simulink model "LoFT_Example3"  (R2024b)
settings: Solver=ode4  StartTime=0.0  StopTime=300  FixedStep=simu.dt  RelTol=1e-3
undefined symbols (not defined in the file): body, circtime, Communication, D1, Delta, irkb, line, LoFT, p0, Pn, s, simu, trip_time, Turbwind, waves, wind
libraries: simulink x350, spsThreePhaseVIMeasurementLib x41, spsThreePhasePISectionLineLib x34, spsThreePhaseParallelRLCLoadLib x21, spsThreePhaseTransformerTwoWindingsLib x14, spsLoadFlowBusLib x10, spsThreePhaseDynamicLoadLib x9, spsSynchronousMachinepuStandardLib x7, spsExcitationSystemLib x7, spsSteamTurbineandGovernorLib x7, spsGenericPowerSystemStabilizerLib x7, spsMultiBandPowerSystemStabilizerLib x7
(part 1 of 49)
settings Model: SimulationMode=accelerator  Creator=85164  LastModifiedBy=85164
settings DataIOCC: ReturnWorkspaceOutputs=off
settings OptimizationCC: ReuseModelBlockBuffer=off
settings RTWCC: GPUComputeCapability=3.5

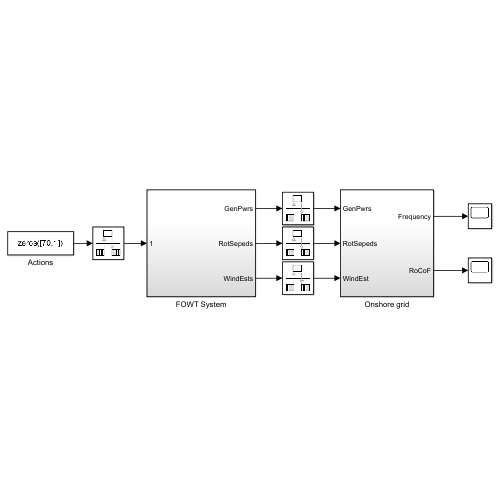
[thumbnail: Simulink's stored preview of the top-level diagram]
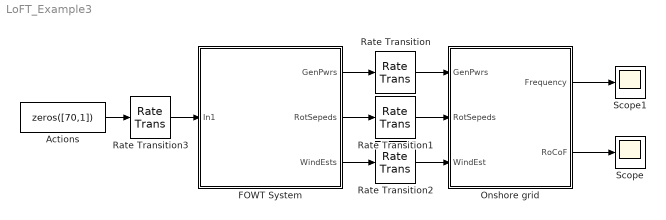
== system LoFT_Example3 ==
  Actions : Constant  Value=zeros([70,1])
  FOWT System : Subsystem
  Onshore grid : Subsystem
  Rate Transition : RateTransition  OutPortSampleTime=simu.grid_dt
  Rate Transition1 : RateTransition  OutPortSampleTime=simu.grid_dt
  Rate Transition2 : RateTransition  OutPortSampleTime=simu.grid_dt
  Rate Transition3 : RateTransition  OutPortSampleTime=simu.turbine_dt
  Scope : Scope
  Scope1 : Scope
  wires:
  FOWT System/1(GenPwrs) -> Rate Transition/1
  FOWT System/2(RotSepeds) -> Rate Transition1/1
  FOWT System/3(WindEsts) -> Rate Transition2/1
  Actions/1 -> Rate Transition3/1
  Onshore grid/1(Frequency) -> Scope1/1
  Onshore grid/2(RoCoF) -> Scope/1
  Rate Transition/1 -> Onshore grid/1(GenPwrs)
  Rate Transition1/1 -> Onshore grid/2(RotSepeds)
  Rate Transition2/1 -> Onshore grid/3(WindEst)
  Rate Transition3/1 -> FOWT System/1(In1)

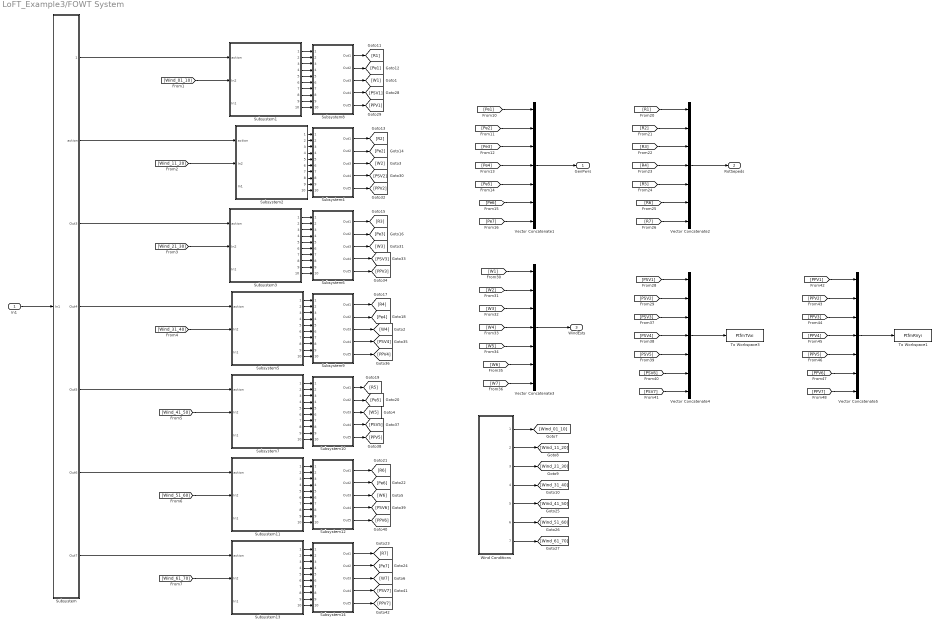
== system LoFT_Example3/FOWT System ==
  In1 : Inport
  Subsystem : Subsystem
  Subsystem1 : Subsystem
  Subsystem10 : Subsystem
  Subsystem11 : Subsystem
  Subsystem12 : Subsystem
  Subsystem13 : Subsystem
  Subsystem14 : Subsystem
  Subsystem2 : Subsystem
  Subsystem3 : Subsystem
  Subsystem4 : Subsystem
  Subsystem5 : Subsystem
  Subsystem6 : Subsystem
  Subsystem7 : Subsystem
  Subsystem8 : Subsystem
  Subsystem9 : Subsystem
  To Workspace1 : ToWorkspace  VariableName=PtfmRVyi  SampleTime=-1
      settings: Save2DSignal=2-D array (concatenate along first dimension)
  To Workspace3 : ToWorkspace  VariableName=PtfmTVxi  SampleTime=-1
      settings: Save2DSignal=2-D array (concatenate along first dimension)
  Vector Concatenate{1..5} (5 alike) : Concatenate  NumInputs=7
  Wind Conditions : Subsystem
  GenPwrs : Outport
  RotSepeds : Outport  Port=2
  WindEsts : Outport  Port=3
  wires:
  [Pe4] -> Vector Concatenate1/4
  [Pe1] -> Vector Concatenate1/1
  [Pe5] -> Vector Concatenate1/5
  [Pe3] -> Vector Concatenate1/3
  [Pe7] -> Vector Concatenate1/7
  [Pe2] -> Vector Concatenate1/2
  [Pe6] -> Vector Concatenate1/6
  [R2] -> Vector Concatenate2/2
  [R3] -> Vector Concatenate2/3
  [R4] -> Vector Concatenate2/4
  [R7] -> Vector Concatenate2/7
  [R5] -> Vector Concatenate2/5
  [R6] -> Vector Concatenate2/6
  [R1] -> Vector Concatenate2/1
  Vector Concatenate1/1 -> GenPwrs/1
  Vector Concatenate2/1 -> RotSepeds/1
  Subsystem/1(1) -> Subsystem1/1(action)
  Vector Concatenate3/1 -> WindEsts/1
  [W5] -> Vector Concatenate3/5
  [W3] -> Vector Concatenate3/3
  [W2] -> Vector Concatenate3/2
  [W1] -> Vector Concatenate3/1
  [W6] -> Vector Concatenate3/6
  [W7] -> Vector Concatenate3/7
  [W4] -> Vector Concatenate3/4
  Wind Conditions/1(1) -> [Wind_01_10]
  Wind Conditions/2(2) -> [Wind_11_20]
  Wind Conditions/3(3) -> [Wind_21_30]
  Wind Conditions/4(4) -> [Wind_31_40]
  Wind Conditions/5(5) -> [Wind_41_50]
  Wind Conditions/6(6) -> [Wind_51_60]
  Wind Conditions/7(7) -> [Wind_61_70]
  [Wind_01_10] -> Subsystem1/2(In2)
  [Wind_11_20] -> Subsystem2/2(In2)
  Subsystem/2(action) -> Subsystem2/1(action)
  [Wind_21_30] -> Subsystem3/2(In2)
  Subsystem/3(Out3) -> Subsystem3/1(action)
  Subsystem/4(Out4) -> Subsystem5/1(action)
  [Wind_31_40] -> Subsystem5/2(In2)
  Subsystem/5(Out5) -> Subsystem7/1(action)
  [Wind_41_50] -> Subsystem7/2(In2)
  Subsystem/6(Out6) -> Subsystem11/1(action)
  [Wind_51_60] -> Subsystem11/2(In2)
  [Wind_61_70] -> Subsystem13/2(In2)
  Subsystem/7(Out7) -> Subsystem13/1(action)
  In1/1 -> Subsystem/1(In1)
  Subsystem4/4(Out4) -> [PSV2]
  Subsystem13/4(4) -> Subsystem14/4(4)
  Subsystem8/3(Out3) -> [W1]
  Subsystem1/10(10) -> Subsystem8/10(10)
  Subsystem12/2(Out2) -> [Pe6]
  Subsystem1/7(7) -> Subsystem8/7(7)
  Subsystem10/2(Out2) -> [Pe5]
  Subsystem12/5(Out5) -> [PPV6]
  Subsystem14/4(Out4) -> [PSV7]
  Subsystem14/2(Out2) -> [Pe7]
  Subsystem4/2(Out2) -> [Pe2]
  Subsystem10/4(Out4) -> [PSV5]
  Subsystem9/2(Out2) -> [Pe4]
  Subsystem11/9(9) -> Subsystem12/9(9)
  Subsystem2/2(2) -> Subsystem4/2(2)
  Subsystem9/4(Out4) -> [PSV4]
  Subsystem13/6(6) -> Subsystem14/6(6)
  Subsystem12/4(Out4) -> [PSV6]
  Subsystem3/8(8) -> Subsystem6/8(8)
  Subsystem7/8(8) -> Subsystem10/8(8)
  Subsystem5/10(10) -> Subsystem9/10(10)
  Subsystem5/7(7) -> Subsystem9/7(7)
  Subsystem4/5(Out5) -> [PPV2]
  Subsystem8/5(Out5) -> [PPV1]
  Subsystem11/4(4) -> Subsystem12/4(4)
  Subsystem9/1(Out1) -> [R4]
  Subsystem4/1(Out1) -> [R2]
  Subsystem6/2(Out2) -> [Pe3]
  Subsystem12/1(Out1) -> [R6]
  Subsystem10/1(Out1) -> [R5]
  Subsystem8/4(Out4) -> [PSV1]
  Subsystem9/3(Out3) -> [W4]
  Subsystem11/6(6) -> Subsystem12/6(6)
  Subsystem14/1(Out1) -> [R7]
  Subsystem5/3(3) -> Subsystem9/3(3)
  Subsystem13/5(5) -> Subsystem14/5(5)
  Subsystem13/9(9) -> Subsystem14/9(9)
  Subsystem6/1(Out1) -> [R3]
  Subsystem11/2(2) -> Subsystem12/2(2)
  Subsystem7/4(4) -> Subsystem10/4(4)
  Subsystem3/4(4) -> Subsystem6/4(4)
  Subsystem11/7(7) -> Subsystem12/7(7)
  Subsystem13/10(10) -> Subsystem14/10(10)
  Subsystem7/2(2) -> Subsystem10/2(2)
  Subsystem2/3(3) -> Subsystem4/3(3)
  Subsystem7/1(1) -> Subsystem10/1(1)
  Subsystem11/10(10) -> Subsystem12/10(10)
  Subsystem7/9(9) -> Subsystem10/9(9)
  Subsystem1/2(2) -> Subsystem8/2(2)
  Subsystem7/3(3) -> Subsystem10/3(3)
  Subsystem5/5(5) -> Subsystem9/5(5)
  Subsystem11/8(8) -> Subsystem12/8(8)
  Subsystem5/8(8) -> Subsystem9/8(8)
  Subsystem3/3(3) -> Subsystem6/3(3)
  Subsystem11/1(1) -> Subsystem12/1(1)
  Subsystem3/5(5) -> Subsystem6/5(5)
  Subsystem5/6(6) -> Subsystem9/6(6)
  Subsystem3/7(7) -> Subsystem6/7(7)
  Subsystem7/7(7) -> Subsystem10/7(7)
  Subsystem8/2(Out2) -> [Pe1]
  Subsystem11/5(5) -> Subsystem12/5(5)
  Subsystem5/4(4) -> Subsystem9/4(4)
  Subsystem6/4(Out4) -> [PSV3]
  Subsystem2/10(10) -> Subsystem4/10(10)
  Subsystem1/8(8) -> Subsystem8/8(8)
  Subsystem5/9(9) -> Subsystem9/9(9)
  Subsystem13/3(3) -> Subsystem14/3(3)
  Subsystem13/2(2) -> Subsystem14/2(2)
  Subsystem10/5(Out5) -> [PPV5]
  Subsystem13/7(7) -> Subsystem14/7(7)
  Subsystem12/3(Out3) -> [W6]
  Subsystem10/3(Out3) -> [W5]
  Subsystem13/8(8) -> Subsystem14/8(8)
  Subsystem3/9(9) -> Subsystem6/9(9)
  Subsystem3/1(1) -> Subsystem6/1(1)
  Subsystem1/6(6) -> Subsystem8/6(6)
  Subsystem2/8(8) -> Subsystem4/8(8)
  Subsystem1/9(9) -> Subsystem8/9(9)
  Subsystem2/4(4) -> Subsystem4/4(4)
  Subsystem2/9(9) -> Subsystem4/9(9)
  Subsystem6/5(Out5) -> [PPV3]
  Subsystem13/1(1) -> Subsystem14/1(1)
  Subsystem3/2(2) -> Subsystem6/2(2)
  Subsystem14/5(Out5) -> [PPV7]
  Subsystem2/1(1) -> Subsystem4/1(1)
  Subsystem14/3(Out3) -> [W7]
  Subsystem11/3(3) -> Subsystem12/3(3)
  Subsystem1/4(4) -> Subsystem8/4(4)
  Subsystem4/3(Out3) -> [W2]
  Subsystem5/2(2) -> Subsystem9/2(2)
  Subsystem2/7(7) -> Subsystem4/7(7)
  Subsystem2/6(6) -> Subsystem4/6(6)
  Subsystem3/6(6) -> Subsystem6/6(6)
  Subsystem5/1(1) -> Subsystem9/1(1)
  Subsystem1/5(5) -> Subsystem8/5(5)
  Subsystem7/10(10) -> Subsystem10/10(10)
  Subsystem8/1(Out1) -> [R1]
  Subsystem9/5(Out5) -> [PPV4]
  Subsystem2/5(5) -> Subsystem4/5(5)
  Subsystem6/3(Out3) -> [W3]
  Subsystem3/10(10) -> Subsystem6/10(10)
  Subsystem1/3(3) -> Subsystem8/3(3)
  Subsystem1/1(1) -> Subsystem8/1(1)
  Subsystem7/6(6) -> Subsystem10/6(6)
  Subsystem7/5(5) -> Subsystem10/5(5)
  [PSV5] -> Vector Concatenate4/5
  [PSV7] -> Vector Concatenate4/7
  Vector Concatenate4/1 -> To Workspace3/1
  [PPV7] -> Vector Concatenate5/7
  [PPV4] -> Vector Concatenate5/4
  [PPV6] -> Vector Concatenate5/6
  [PSV2] -> Vector Concatenate4/2
  [PSV6] -> Vector Concatenate4/6
  [PSV3] -> Vector Concatenate4/3
  [PPV2] -> Vector Concatenate5/2
  [PSV4] -> Vector Concatenate4/4
  [PPV5] -> Vector Concatenate5/5
  [PPV3] -> Vector Concatenate5/3
  [PPV1] -> Vector Concatenate5/1
  Vector Concatenate5/1 -> To Workspace1/1
  [PSV1] -> Vector Concatenate4/1

== system LoFT_Example3/Onshore grid ==
  GenPwrs : Inport
  RotSepeds : Inport  Port=2
  WindEst : Inport  Port=3
  Monitor : Subsystem
  Onshore Grid : Subsystem
  Frequency : Outport
  RoCoF : Outport  Port=2
  wires:
  RotSepeds/1 -> Monitor/2(RotSepeds)
  WindEst/1 -> Monitor/3(3)
  Onshore Grid/1(Frequency) -> Frequency/1
  Onshore Grid/2(RoCoF) -> RoCoF/1
  GenPwrs/1 -> Onshore Grid/1(1), Monitor/1(GenPwrs)

== system LoFT_Example3/FOWT System/Subsystem ==
  In1 : Inport
  Demux : Demux  Outputs=70
  Mux{,1..6} (7 alike) : Mux  Inputs=10
  1 : Outport
  action : Outport  Port=2
  Out3 : Outport  Port=3
  Out4 : Outport  Port=4
  Out5 : Outport  Port=5
  Out6 : Outport  Port=6
  Out7 : Outport  Port=7
  wires:
  Demux/25 -> Mux2/5
  Demux/42 -> Mux4/2
  Demux/37 -> Mux3/7
  Demux/6 -> Mux/6
  Demux/56 -> Mux5/6
  Demux/9 -> Mux/9
  Demux/36 -> Mux3/6
  Demux/52 -> Mux5/2
  Demux/67 -> Mux6/7
  Demux/13 -> Mux1/3
  Demux/61 -> Mux6/1
  Demux/55 -> Mux5/5
  Demux/47 -> Mux4/7
  Demux/8 -> Mux/8
  Demux/29 -> Mux2/9
  Demux/7 -> Mux/7
  Demux/68 -> Mux6/8
  Demux/59 -> Mux5/9
  Demux/60 -> Mux5/10
  Demux/39 -> Mux3/9
  Demux/58 -> Mux5/8
  Demux/62 -> Mux6/2
  Demux/53 -> Mux5/3
  Demux/20 -> Mux1/10
  Demux/54 -> Mux5/4
  Demux/23 -> Mux2/3
  Demux/51 -> Mux5/1
  Mux3/1 -> Out4/1
  Demux/38 -> Mux3/8
  Demux/57 -> Mux5/7
  Demux/63 -> Mux6/3
  Demux/27 -> Mux2/7
  Demux/15 -> Mux1/5
  Demux/19 -> Mux1/9
  Demux/49 -> Mux4/9
  Demux/28 -> Mux2/8
  Demux/32 -> Mux3/2
  Demux/65 -> Mux6/5
  Demux/43 -> Mux4/3
  Demux/45 -> Mux4/5
  Demux/41 -> Mux4/1
  Demux/11 -> Mux1/1
  Demux/30 -> Mux2/10
  Demux/46 -> Mux4/6
  Mux/1 -> 1/1
  Demux/5 -> Mux/5
  Demux/40 -> Mux3/10
  Demux/2 -> Mux/2
  Demux/44 -> Mux4/4
  Demux/3 -> Mux/3
  Demux/48 -> Mux4/8
  Demux/50 -> Mux4/10
  Demux/24 -> Mux2/4
  Demux/21 -> Mux2/1
  Demux/22 -> Mux2/2
  Demux/26 -> Mux2/6
  Mux6/1 -> Out7/1
  Demux/12 -> Mux1/2
  Demux/35 -> Mux3/5
  Demux/31 -> Mux3/1
  Demux/4 -> Mux/4
  Demux/33 -> Mux3/3
  Demux/34 -> Mux3/4
  Demux/10 -> Mux/10
  Demux/64 -> Mux6/4
  Demux/66 -> Mux6/6
  Demux/70 -> Mux6/10
  Demux/69 -> Mux6/9
  Demux/14 -> Mux1/4
  Demux/16 -> Mux1/6
  Demux/17 -> Mux1/7
  Demux/18 -> Mux1/8
  Demux/1 -> Mux/1
  Mux1/1 -> action/1
  Mux2/1 -> Out3/1
  Mux5/1 -> Out6/1
  Mux4/1 -> Out5/1
  In1/1 -> Demux/1

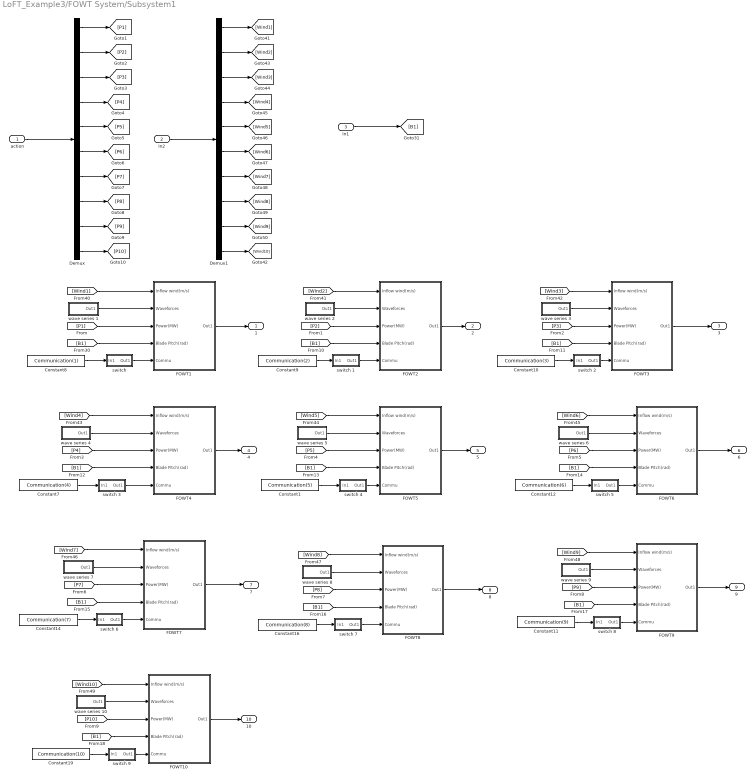
== system LoFT_Example3/FOWT System/Subsystem1 ==
  action : Inport
  In2 : Inport  Port=2
  In1 : Inport  Port=3
  Constant1 : Constant  Value=Communication(5)
  Constant10 : Constant  Value=Communication(3)
  Constant11 : Constant  Value=Communication(9)
  Constant12 : Constant  Value=Communication(6)
  Constant14 : Constant  Value=Communication(7)
  Constant16 : Constant  Value=Communication(8)
  Constant19 : Constant  Value=Communication(10)
  Constant7 : Constant  Value=Communication(4)
  Constant8 : Constant  Value=Communication(1)
  Constant9 : Constant  Value=Communication(2)
  Demux : Demux  Outputs=10
  Demux1 : Demux  Outputs=10
  FOWT1 : Subsystem  mask{Aero=LoFT.Aero, Hydro=LoFT.Hydro, Mooring=LoFT.Mooring, Property=LoFT.Property, Controller=LoFT.Controller, Initposition=[15,  0,  3*pi/180], Initstate=[6.8*pi/30, 9]}
      mask prompts: Aero "Aerodynamics"; Hydro "Hydrodynamics"; Mooring "Mooring lookup table"; Property "Hull mass, inertia and volume"; Controller "Local controller"; Initposition "Initial Hull position"; Initstate "Initial RotSpeed and WindEst"
      mask DialogControl DescGroupVar Prompt: LoFT
      mask DialogControl FOWT Prompt: Low-order modelling of floating offshore wind turbine for training
      mask DialogControl Manuscript Prompt: Citation
      mask DialogControl scriptname Prompt: Primary Frequency Response of Floating Offshore Wind Turbines via Deep Reinforcement Learning and Domain Randomization
      mask DialogControl ParameterGroupVar Prompt: 参数
  FOWT10 : Subsystem  mask{Aero=LoFT.Aero, Hydro=LoFT.Hydro, Mooring=LoFT.Mooring, Property=LoFT.Property, Controller=LoFT.Controller, Initposition=[5,  0,  3*pi/180], Initstate=[6.8*pi/30, 9]}
      mask prompts: Aero "Aerodynamics"; Hydro "Hydrodynamics"; Mooring "Mooring lookup table"; Property "Hull mass, inertia and volume"; Controller "Local controller"; Initposition "Initial Hull position"; Initstate "Initial RotSpeed and WindEst"
      mask DialogControl DescGroupVar Prompt: LoFT
      mask DialogControl FOWT Prompt: Low-order modelling of floating offshore wind turbine for training
      mask DialogControl Manuscript Prompt: Citation
      mask DialogControl scriptname Prompt: Primary Frequency Response of Floating Offshore Wind Turbines via Deep Reinforcement Learning and Domain Randomization
      mask DialogControl ParameterGroupVar Prompt: 参数
  FOWT2 : Subsystem  mask{Aero=LoFT.Aero, Hydro=LoFT.Hydro, Mooring=LoFT.Mooring, Property=LoFT.Property, Controller=LoFT.Controller, Initposition=[40,  0,  3*pi/180], Initstate=[6.8*pi/30, 9]}
      mask prompts: Aero "Aerodynamics"; Hydro "Hydrodynamics"; Mooring "Mooring lookup table"; Property "Hull mass, inertia and volume"; Controller "Local controller"; Initposition "Initial Hull position"; Initstate "Initial RotSpeed and WindEst"
      mask DialogControl DescGroupVar Prompt: LoFT
      mask DialogControl FOWT Prompt: Low-order modelling of floating offshore wind turbine for training
      mask DialogControl Manuscript Prompt: Citation
      mask DialogControl scriptname Prompt: Primary Frequency Response of Floating Offshore Wind Turbines via Deep Reinforcement Learning and Domain Randomization
      mask DialogControl ParameterGroupVar Prompt: 参数
  FOWT3 : Subsystem  mask{Aero=LoFT.Aero, Hydro=LoFT.Hydro, Mooring=LoFT.Mooring, Property=LoFT.Property, Controller=LoFT.Controller, Initposition=[25,  0,  3*pi/180], Initstate=[6.8*pi/30, 9]}
      mask prompts: Aero "Aerodynamics"; Hydro "Hydrodynamics"; Mooring "Mooring lookup table"; Property "Hull mass, inertia and volume"; Controller "Local controller"; Initposition "Initial Hull position"; Initstate "Initial RotSpeed and WindEst"
      mask DialogControl DescGroupVar Prompt: LoFT
      mask DialogControl FOWT Prompt: Low-order modelling of floating offshore wind turbine for training
      mask DialogControl Manuscript Prompt: Citation
      mask DialogControl scriptname Prompt: Primary Frequency Response of Floating Offshore Wind Turbines via Deep Reinforcement Learning and Domain Randomization
      mask DialogControl ParameterGroupVar Prompt: 参数
  FOWT4 : Subsystem  mask{Aero=LoFT.Aero, Hydro=LoFT.Hydro, Mooring=LoFT.Mooring, Property=LoFT.Property, Controller=LoFT.Controller, Initposition=[15,  0,  3*pi/180], Initstate=[6.8*pi/30, 9]}
      mask prompts: Aero "Aerodynamics"; Hydro "Hydrodynamics"; Mooring "Mooring lookup table"; Property "Hull mass, inertia and volume"; Controller "Local controller"; Initposition "Initial Hull position"; Initstate "Initial RotSpeed and WindEst"
      mask DialogControl DescGroupVar Prompt: LoFT
      mask DialogControl FOWT Prompt: Low-order modelling of floating offshore wind turbine for training
      mask DialogControl Manuscript Prompt: Citation
      mask DialogControl scriptname Prompt: Primary Frequency Response of Floating Offshore Wind Turbines via Deep Reinforcement Learning and Domain Randomization
      mask DialogControl ParameterGroupVar Prompt: 参数
  FOWT5 : Subsystem  mask{Aero=LoFT.Aero, Hydro=LoFT.Hydro, Mooring=LoFT.Mooring, Property=LoFT.Property, Controller=LoFT.Controller, Initposition=[40,  0,  3*pi/180], Initstate=[6.8*pi/30, 9]}
      mask prompts: Aero "Aerodynamics"; Hydro "Hydrodynamics"; Mooring "Mooring lookup table"; Property "Hull mass, inertia and volume"; Controller "Local controller"; Initposition "Initial Hull position"; Initstate "Initial RotSpeed and WindEst"
      mask DialogControl DescGroupVar Prompt: LoFT
      mask DialogControl FOWT Prompt: Low-order modelling of floating offshore wind turbine for training
      mask DialogControl Manuscript Prompt: Citation
      mask DialogControl scriptname Prompt: Primary Frequency Response of Floating Offshore Wind Turbines via Deep Reinforcement Learning and Domain Randomization
      mask DialogControl ParameterGroupVar Prompt: 参数
  FOWT6 : Subsystem  mask{Aero=LoFT.Aero, Hydro=LoFT.Hydro, Mooring=LoFT.Mooring, Property=LoFT.Property, Controller=LoFT.Controller, Initposition=[25,  0,  3*pi/180], Initstate=[6.8*pi/30, 9]}
      mask prompts: Aero "Aerodynamics"; Hydro "Hydrodynamics"; Mooring "Mooring lookup table"; Property "Hull mass, inertia and volume"; Controller "Local controller"; Initposition "Initial Hull position"; Initstate "Initial RotSpeed and WindEst"
      mask DialogControl DescGroupVar Prompt: LoFT
      mask DialogControl FOWT Prompt: Low-order modelling of floating offshore wind turbine for training
      mask DialogControl Manuscript Prompt: Citation
      mask DialogControl scriptname Prompt: Primary Frequency Response of Floating Offshore Wind Turbines via Deep Reinforcement Learning and Domain Randomization
      mask DialogControl ParameterGroupVar Prompt: 参数
  FOWT7 : Subsystem  mask{Aero=LoFT.Aero, Hydro=LoFT.Hydro, Mooring=LoFT.Mooring, Property=LoFT.Property, Controller=LoFT.Controller, Initposition=[15,  0,  3*pi/180], Initstate=[6.8*pi/30, 9]}
      mask prompts: Aero "Aerodynamics"; Hydro "Hydrodynamics"; Mooring "Mooring lookup table"; Property "Hull mass, inertia and volume"; Controller "Local controller"; Initposition "Initial Hull position"; Initstate "Initial RotSpeed and WindEst"
      mask DialogControl DescGroupVar Prompt: LoFT
      mask DialogControl FOWT Prompt: Low-order modelling of floating offshore wind turbine for training
      mask DialogControl Manuscript Prompt: Citation
      mask DialogControl scriptname Prompt: Primary Frequency Response of Floating Offshore Wind Turbines via Deep Reinforcement Learning and Domain Randomization
      mask DialogControl ParameterGroupVar Prompt: 参数
  FOWT8 : Subsystem  mask{Aero=LoFT.Aero, Hydro=LoFT.Hydro, Mooring=LoFT.Mooring, Property=LoFT.Property, Controller=LoFT.Controller, Initposition=[40,  0,  3*pi/180], Initstate=[6.8*pi/30, 9]}
      mask prompts: Aero "Aerodynamics"; Hydro "Hydrodynamics"; Mooring "Mooring lookup table"; Property "Hull mass, inertia and volume"; Controller "Local controller"; Initposition "Initial Hull position"; Initstate "Initial RotSpeed and WindEst"
      mask DialogControl DescGroupVar Prompt: LoFT
      mask DialogControl FOWT Prompt: Low-order modelling of floating offshore wind turbine for training
      mask DialogControl Manuscript Prompt: Citation
      mask DialogControl scriptname Prompt: Primary Frequency Response of Floating Offshore Wind Turbines via Deep Reinforcement Learning and Domain Randomization
      mask DialogControl ParameterGroupVar Prompt: 参数
  FOWT9 : Subsystem  mask{Aero=LoFT.Aero, Hydro=LoFT.Hydro, Mooring=LoFT.Mooring, Property=LoFT.Property, Controller=LoFT.Controller, Initposition=[25,  0,  3*pi/180], Initstate=[6.8*pi/30, 9]}
      mask prompts: Aero "Aerodynamics"; Hydro "Hydrodynamics"; Mooring "Mooring lookup table"; Property "Hull mass, inertia and volume"; Controller "Local controller"; Initposition "Initial Hull position"; Initstate "Initial RotSpeed and WindEst"
      mask DialogControl DescGroupVar Prompt: LoFT
      mask DialogControl FOWT Prompt: Low-order modelling of floating offshore wind turbine for training
      mask DialogControl Manuscript Prompt: Citation
      mask DialogControl scriptname Prompt: Primary Frequency Response of Floating Offshore Wind Turbines via Deep Reinforcement Learning and Domain Randomization
      mask DialogControl ParameterGroupVar Prompt: 参数
  "switch " : Subsystem
  switch 1 : Subsystem
  switch 2 : Subsystem
  switch 3 : Subsystem
  switch 4 : Subsystem
  switch 5 : Subsystem
  switch 6 : Subsystem
  switch 7 : Subsystem
  switch 8 : Subsystem
  switch 9 : Subsystem
  wave series 1 : Subsystem
  wave series 10 : Subsystem
  wave series 2 : Subsystem
  wave series 3 : Subsystem
  wave series 4 : Subsystem
  wave series 5 : Subsystem
  wave series 6 : Subsystem
  wave series 7 : Subsystem
  wave series 8 : Subsystem
  wave series 9 : Subsystem
  1 : Outport
  2 : Outport  Port=2
  3 : Outport  Port=3
  4 : Outport  Port=4
  5 : Outport  Port=5
  6 : Outport  Port=6
  7 : Outport  Port=7
  8 : Outport  Port=8
  9 : Outport  Port=9
  10 : Outport  Port=10
  wires:
  Demux/9 -> [P9]
  Demux/10 -> [P10]
  wave series 10/1(Out1) -> FOWT10/2(Waveforces)
  [B1] -> FOWT10/4(Blade Pitch(rad))
  Constant19/1 -> switch 9/1(In1)
  switch 9/1(Out1) -> FOWT10/5(Commu)
  [P10] -> FOWT10/3(Power(MW))
  [Wind10] -> FOWT10/1(Inflow wind(m/s))
  Constant11/1 -> switch 8/1(In1)
  [P9] -> FOWT9/3(Power(MW))
  [B1] -> FOWT9/4(Blade Pitch(rad))
  [Wind9] -> FOWT9/1(Inflow wind(m/s))
  switch 8/1(Out1) -> FOWT9/5(Commu)
  wave series 9/1(Out1) -> FOWT9/2(Waveforces)
  Demux/6 -> [P6]
  Demux/7 -> [P7]
  Demux/8 -> [P8]
  Demux/5 -> [P5]
  Demux/1 -> [P1]
  Demux/4 -> [P4]
  action/1 -> Demux/1
  Demux/3 -> [P3]
  Demux/2 -> [P2]
  [Wind2] -> FOWT2/1(Inflow wind(m/s))
  wave series 2/1(Out1) -> FOWT2/2(Waveforces)
  [Wind4] -> FOWT4/1(Inflow wind(m/s))
  wave series 8/1(Out1) -> FOWT8/2(Waveforces)
  [Wind3] -> FOWT3/1(Inflow wind(m/s))
  switch 4/1(Out1) -> FOWT5/5(Commu)
  switch 7/1(Out1) -> FOWT8/5(Commu)
  wave series 4/1(Out1) -> FOWT4/2(Waveforces)
  switch 6/1(Out1) -> FOWT7/5(Commu)
  Constant16/1 -> switch 7/1(In1)
  wave series 6/1(Out1) -> FOWT6/2(Waveforces)
  [Wind8] -> FOWT8/1(Inflow wind(m/s))
  wave series 1/1(Out1) -> FOWT1/2(Waveforces)
  [Wind5] -> FOWT5/1(Inflow wind(m/s))
  Constant8/1 -> "switch "/1(In1)
  "switch "/1(Out1) -> FOWT1/5(Commu)
  [P8] -> FOWT8/3(Power(MW))
  [B1] -> FOWT8/4(Blade Pitch(rad))
  wave series 5/1(Out1) -> FOWT5/2(Waveforces)
  Constant10/1 -> switch 2/1(In1)
  [P5] -> FOWT5/3(Power(MW))
  Constant14/1 -> switch 6/1(In1)
  [P6] -> FOWT6/3(Power(MW))
  Constant12/1 -> switch 5/1(In1)
  [P4] -> FOWT4/3(Power(MW))
  wave series 7/1(Out1) -> FOWT7/2(Waveforces)
  [Wind7] -> FOWT7/1(Inflow wind(m/s))
  [P1] -> FOWT1/3(Power(MW))
  [B1] -> FOWT7/4(Blade Pitch(rad))
  [P3] -> FOWT3/3(Power(MW))
  Constant1/1 -> switch 4/1(In1)
  switch 1/1(Out1) -> FOWT2/5(Commu)
  [Wind1] -> FOWT1/1(Inflow wind(m/s))
  [P2] -> FOWT2/3(Power(MW))
  [Wind6] -> FOWT6/1(Inflow wind(m/s))
  wave series 3/1(Out1) -> FOWT3/2(Waveforces)
  Constant7/1 -> switch 3/1(In1)
  Constant9/1 -> switch 1/1(In1)
  [P7] -> FOWT7/3(Power(MW))
  switch 5/1(Out1) -> FOWT6/5(Commu)
  switch 3/1(Out1) -> FOWT4/5(Commu)
  switch 2/1(Out1) -> FOWT3/5(Commu)
  Demux1/4 -> [Wind4]
  In2/1 -> Demux1/1
  Demux1/7 -> [Wind7]
  Demux1/8 -> [Wind8]
  Demux1/3 -> [Wind3]
  Demux1/2 -> [Wind2]
  Demux1/5 -> [Wind5]
  Demux1/9 -> [Wind9]
  Demux1/10 -> [Wind10]
  Demux1/1 -> [Wind1]
  Demux1/6 -> [Wind6]
  FOWT1/1(Out1) -> 1/1
  FOWT2/1(Out1) -> 2/1
  FOWT3/1(Out1) -> 3/1
  FOWT4/1(Out1) -> 4/1
  FOWT5/1(Out1) -> 5/1
  FOWT6/1(Out1) -> 6/1
  FOWT7/1(Out1) -> 7/1
  FOWT8/1(Out1) -> 8/1
  FOWT9/1(Out1) -> 9/1
  FOWT10/1(Out1) -> 10/1
  In1/1 -> [B1]
  [B1] -> FOWT1/4(Blade Pitch(rad))
  [B1] -> FOWT2/4(Blade Pitch(rad))
  [B1] -> FOWT3/4(Blade Pitch(rad))
  [B1] -> FOWT4/4(Blade Pitch(rad))
  [B1] -> FOWT5/4(Blade Pitch(rad))
  [B1] -> FOWT6/4(Blade Pitch(rad))

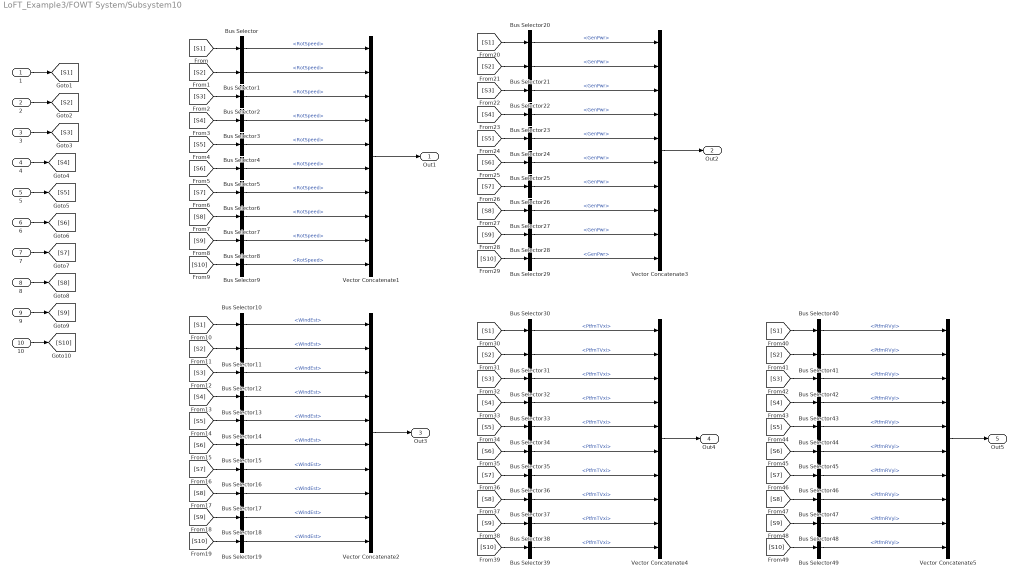
== system LoFT_Example3/FOWT System/Subsystem10 ==
  1 : Inport
  2 : Inport  Port=2
  3 : Inport  Port=3
  4 : Inport  Port=4
  5 : Inport  Port=5
  6 : Inport  Port=6
  7 : Inport  Port=7
  8 : Inport  Port=8
  9 : Inport  Port=9
  10 : Inport  Port=10
  Bus Selector{,1..9} (10 alike) : BusSelector  OutputSignals=RotSpeed
  Bus Selector{10..19} (10 alike) : BusSelector  OutputSignals=WindEst
  Bus Selector{20..29} (10 alike) : BusSelector  OutputSignals=GenPwr
  Bus Selector{30..39} (10 alike) : BusSelector  OutputSignals=PtfmTVxi
  Bus Selector{40..49} (10 alike) : BusSelector  OutputSignals=PtfmRVyi
  Vector Concatenate{1..5} (5 alike) : Concatenate  NumInputs=10
  Out1 : Outport
  Out2 : Outport  Port=2
  Out3 : Outport  Port=3
  Out4 : Outport  Port=4
  Out5 : Outport  Port=5
  wires:
  1/1 -> [S1]
  2/1 -> [S2]
  3/1 -> [S3]
  4/1 -> [S4]
  5/1 -> [S5]
  6/1 -> [S6]
  7/1 -> [S7]
  8/1 -> [S8]
  9/1 -> [S9]
  10/1 -> [S10]
  [S1] -> Bus Selector/1
  Vector Concatenate1/1 -> Out1/1
  Bus Selector/1 -> Vector Concatenate1/1  "<RotSpeed>"
  [S2] -> Bus Selector1/1
  Bus Selector1/1 -> Vector Concatenate1/2  "<RotSpeed>"
  Bus Selector2/1 -> Vector Concatenate1/3  "<RotSpeed>"
  [S3] -> Bus Selector2/1
  [S4] -> Bus Selector3/1
  Bus Selector3/1 -> Vector Concatenate1/4  "<RotSpeed>"
  [S5] -> Bus Selector4/1
  [S6] -> Bus Selector5/1
  [S7] -> Bus Selector6/1
  [S8] -> Bus Selector7/1
  [S9] -> Bus Selector8/1
  [S10] -> Bus Selector9/1
  Bus Selector4/1 -> Vector Concatenate1/5  "<RotSpeed>"
  Bus Selector5/1 -> Vector Concatenate1/6  "<RotSpeed>"
  Bus Selector6/1 -> Vector Concatenate1/7  "<RotSpeed>"
  Bus Selector7/1 -> Vector Concatenate1/8  "<RotSpeed>"
  Bus Selector8/1 -> Vector Concatenate1/9  "<RotSpeed>"
  Bus Selector9/1 -> Vector Concatenate1/10  "<RotSpeed>"
  Bus Selector19/1 -> Vector Concatenate2/10  "<WindEst>"
  Bus Selector18/1 -> Vector Concatenate2/9  "<WindEst>"
  Bus Selector17/1 -> Vector Concatenate2/8  "<WindEst>"
  Bus Selector16/1 -> Vector Concatenate2/7  "<WindEst>"
  Bus Selector15/1 -> Vector Concatenate2/6  "<WindEst>"
  Bus Selector14/1 -> Vector Concatenate2/5  "<WindEst>"
  [S10] -> Bus Selector19/1
  [S9] -> Bus Selector18/1
  [S7] -> Bus Selector16/1
  [S6] -> Bus Selector15/1
  [S5] -> Bus Selector14/1
  Bus Selector13/1 -> Vector Concatenate2/4  "<WindEst>"
  [S4] -> Bus Selector13/1
  [S3] -> Bus Selector12/1
  Bus Selector12/1 -> Vector Concatenate2/3  "<WindEst>"
  Bus Selector11/1 -> Vector Concatenate2/2  "<WindEst>"
  [S2] -> Bus Selector11/1
  Bus Selector10/1 -> Vector Concatenate2/1  "<WindEst>"
  [S1] -> Bus Selector10/1
  [S1] -> Bus Selector20/1
  Bus Selector20/1 -> Vector Concatenate3/1  "<GenPwr>"
  [S2] -> Bus Selector21/1
  Bus Selector21/1 -> Vector Concatenate3/2  "<GenPwr>"
  Bus Selector22/1 -> Vector Concatenate3/3  "<GenPwr>"
  [S3] -> Bus Selector22/1
  [S4] -> Bus Selector23/1
  Bus Selector23/1 -> Vector Concatenate3/4  "<GenPwr>"
  [S5] -> Bus Selector24/1
  [S6] -> Bus Selector25/1
  [S7] -> Bus Selector26/1
  [S8] -> Bus Selector27/1
  [S9] -> Bus Selector28/1
  [S10] -> Bus Selector29/1
  Bus Selector24/1 -> Vector Concatenate3/5  "<GenPwr>"
  Bus Selector25/1 -> Vector Concatenate3/6  "<GenPwr>"
  Bus Selector26/1 -> Vector Concatenate3/7  "<GenPwr>"
  Bus Selector27/1 -> Vector Concatenate3/8  "<GenPwr>"
  Bus Selector28/1 -> Vector Concatenate3/9  "<GenPwr>"
  Bus Selector29/1 -> Vector Concatenate3/10  "<GenPwr>"
  [S8] -> Bus Selector17/1
  Vector Concatenate3/1 -> Out2/1
  Vector Concatenate2/1 -> Out3/1
  [S1] -> Bus Selector30/1
  Bus Selector30/1 -> Vector Concatenate4/1  "<PtfmTVxi>"
  Vector Concatenate4/1 -> Out4/1
  [S5] -> Bus Selector44/1
  Bus Selector47/1 -> Vector Concatenate5/8  "<PtfmRVyi>"
  [S1] -> Bus Selector40/1
  Bus Selector40/1 -> Vector Concatenate5/1  "<PtfmRVyi>"
  [S2] -> Bus Selector41/1
  [S4] -> Bus Selector43/1
  [S3] -> Bus Selector42/1
  Bus Selector42/1 -> Vector Concatenate5/3  "<PtfmRVyi>"
  Bus Selector44/1 -> Vector Concatenate5/5  "<PtfmRVyi>"
  Bus Selector43/1 -> Vector Concatenate5/4  "<PtfmRVyi>"
  [S9] -> Bus Selector48/1
  Bus Selector45/1 -> Vector Concatenate5/6  "<PtfmRVyi>"
  Bus Selector48/1 -> Vector Concatenate5/9  "<PtfmRVyi>"
  [S6] -> Bus Selector45/1
  [S10] -> Bus Selector49/1
  Bus Selector49/1 -> Vector Concatenate5/10  "<PtfmRVyi>"
  Vector Concatenate5/1 -> Out5/1
  [S7] -> Bus Selector46/1
  Bus Selector46/1 -> Vector Concatenate5/7  "<PtfmRVyi>"
  Bus Selector41/1 -> Vector Concatenate5/2  "<PtfmRVyi>"
  [S8] -> Bus Selector47/1
  Bus Selector31/1 -> Vector Concatenate4/2  "<PtfmTVxi>"
  [S2] -> Bus Selector31/1
  Bus Selector32/1 -> Vector Concatenate4/3  "<PtfmTVxi>"
  [S3] -> Bus Selector32/1
  [S4] -> Bus Selector33/1
  Bus Selector33/1 -> Vector Concatenate4/4  "<PtfmTVxi>"
  [S5] -> Bus Selector34/1
  Bus Selector34/1 -> Vector Concatenate4/5  "<PtfmTVxi>"
  [S6] -> Bus Selector35/1
  Bus Selector35/1 -> Vector Concatenate4/6  "<PtfmTVxi>"
  [S7] -> Bus Selector36/1
  Bus Selector36/1 -> Vector Concatenate4/7  "<PtfmTVxi>"
  [S8] -> Bus Selector37/1
  Bus Selector37/1 -> Vector Concatenate4/8  "<PtfmTVxi>"
  [S9] -> Bus Selector38/1
  Bus Selector38/1 -> Vector Concatenate4/9  "<PtfmTVxi>"
  [S10] -> Bus Selector39/1
  Bus Selector39/1 -> Vector Concatenate4/10  "<PtfmTVxi>"

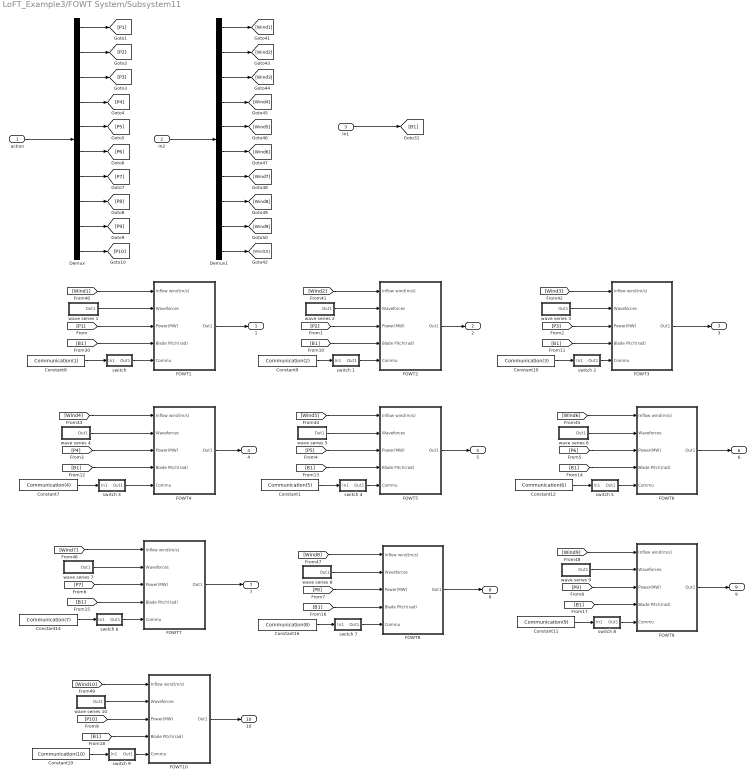
== system LoFT_Example3/FOWT System/Subsystem11 ==
  action : Inport
  In2 : Inport  Port=2
  In1 : Inport  Port=3
  Constant1 : Constant  Value=Communication(5)
  Constant10 : Constant  Value=Communication(3)
  Constant11 : Constant  Value=Communication(9)
  Constant12 : Constant  Value=Communication(6)
  Constant14 : Constant  Value=Communication(7)
  Constant16 : Constant  Value=Communication(8)
  Constant19 : Constant  Value=Communication(10)
  Constant7 : Constant  Value=Communication(4)
  Constant8 : Constant  Value=Communication(1)
  Constant9 : Constant  Value=Communication(2)
  Demux : Demux  Outputs=10
  Demux1 : Demux  Outputs=10
  FOWT1 : Subsystem  mask{Aero=LoFT.Aero, Hydro=LoFT.Hydro, Mooring=LoFT.Mooring, Property=LoFT.Property, Controller=LoFT.Controller, Initposition=[15,  0,  3*pi/180], Initstate=[6.8*pi/30, 9]}
      mask prompts: Aero "Aerodynamics"; Hydro "Hydrodynamics"; Mooring "Mooring lookup table"; Property "Hull mass, inertia and volume"; Controller "Local controller"; Initposition "Initial Hull position"; Initstate "Initial RotSpeed and WindEst"
      mask DialogControl DescGroupVar Prompt: LoFT
      mask DialogControl FOWT Prompt: Low-order modelling of floating offshore wind turbine for training
      mask DialogControl Manuscript Prompt: Citation
      mask DialogControl scriptname Prompt: Primary Frequency Response of Floating Offshore Wind Turbines via Deep Reinforcement Learning and Domain Randomization
      mask DialogControl ParameterGroupVar Prompt: 参数
  FOWT10 : Subsystem  mask{Aero=LoFT.Aero, Hydro=LoFT.Hydro, Mooring=LoFT.Mooring, Property=LoFT.Property, Controller=LoFT.Controller, Initposition=[5,  0,  3*pi/180], Initstate=[6.8*pi/30, 9]}
      mask prompts: Aero "Aerodynamics"; Hydro "Hydrodynamics"; Mooring "Mooring lookup table"; Property "Hull mass, inertia and volume"; Controller "Local controller"; Initposition "Initial Hull position"; Initstate "Initial RotSpeed and WindEst"
      mask DialogControl DescGroupVar Prompt: LoFT
      mask DialogControl FOWT Prompt: Low-order modelling of floating offshore wind turbine for training
      mask DialogControl Manuscript Prompt: Citation
      mask DialogControl scriptname Prompt: Primary Frequency Response of Floating Offshore Wind Turbines via Deep Reinforcement Learning and Domain Randomization
      mask DialogControl ParameterGroupVar Prompt: 参数
  FOWT2 : Subsystem  mask{Aero=LoFT.Aero, Hydro=LoFT.Hydro, Mooring=LoFT.Mooring, Property=LoFT.Property, Controller=LoFT.Controller, Initposition=[40,  0,  3*pi/180], Initstate=[6.8*pi/30, 9]}
      mask prompts: Aero "Aerodynamics"; Hydro "Hydrodynamics"; Mooring "Mooring lookup table"; Property "Hull mass, inertia and volume"; Controller "Local controller"; Initposition "Initial Hull position"; Initstate "Initial RotSpeed and WindEst"
      mask DialogControl DescGroupVar Prompt: LoFT
      mask DialogControl FOWT Prompt: Low-order modelling of floating offshore wind turbine for training
      mask DialogControl Manuscript Prompt: Citation
      mask DialogControl scriptname Prompt: Primary Frequency Response of Floating Offshore Wind Turbines via Deep Reinforcement Learning and Domain Randomization
      mask DialogControl ParameterGroupVar Prompt: 参数
  FOWT3 : Subsystem  mask{Aero=LoFT.Aero, Hydro=LoFT.Hydro, Mooring=LoFT.Mooring, Property=LoFT.Property, Controller=LoFT.Controller, Initposition=[25,  0,  3*pi/180], Initstate=[6.8*pi/30, 9]}
      mask prompts: Aero "Aerodynamics"; Hydro "Hydrodynamics"; Mooring "Mooring lookup table"; Property "Hull mass, inertia and volume"; Controller "Local controller"; Initposition "Initial Hull position"; Initstate "Initial RotSpeed and WindEst"
      mask DialogControl DescGroupVar Prompt: LoFT
      mask DialogControl FOWT Prompt: Low-order modelling of floating offshore wind turbine for training
      mask DialogControl Manuscript Prompt: Citation
      mask DialogControl scriptname Prompt: Primary Frequency Response of Floating Offshore Wind Turbines via Deep Reinforcement Learning and Domain Randomization
      mask DialogControl ParameterGroupVar Prompt: 参数
  FOWT4 : Subsystem  mask{Aero=LoFT.Aero, Hydro=LoFT.Hydro, Mooring=LoFT.Mooring, Property=LoFT.Property, Controller=LoFT.Controller, Initposition=[15,  0,  3*pi/180], Initstate=[6.8*pi/30, 9]}
      mask prompts: Aero "Aerodynamics"; Hydro "Hydrodynamics"; Mooring "Mooring lookup table"; Property "Hull mass, inertia and volume"; Controller "Local controller"; Initposition "Initial Hull position"; Initstate "Initial RotSpeed and WindEst"
      mask DialogControl DescGroupVar Prompt: LoFT
      mask DialogControl FOWT Prompt: Low-order modelling of floating offshore wind turbine for training
      mask DialogControl Manuscript Prompt: Citation
      mask DialogControl scriptname Prompt: Primary Frequency Response of Floating Offshore Wind Turbines via Deep Reinforcement Learning and Domain Randomization
      mask DialogControl ParameterGroupVar Prompt: 参数
  FOWT5 : Subsystem  mask{Aero=LoFT.Aero, Hydro=LoFT.Hydro, Mooring=LoFT.Mooring, Property=LoFT.Property, Controller=LoFT.Controller, Initposition=[40,  0,  3*pi/180], Initstate=[6.8*pi/30, 9]}
      mask prompts: Aero "Aerodynamics"; Hydro "Hydrodynamics"; Mooring "Mooring lookup table"; Property "Hull mass, inertia and volume"; Controller "Local controller"; Initposition "Initial Hull position"; Initstate "Initial RotSpeed and WindEst"
      mask DialogControl DescGroupVar Prompt: LoFT
      mask DialogControl FOWT Prompt: Low-order modelling of floating offshore wind turbine for training
      mask DialogControl Manuscript Prompt: Citation
      mask DialogControl scriptname Prompt: Primary Frequency Response of Floating Offshore Wind Turbines via Deep Reinforcement Learning and Domain Randomization
      mask DialogControl ParameterGroupVar Prompt: 参数
  FOWT6 : Subsystem  mask{Aero=LoFT.Aero, Hydro=LoFT.Hydro, Mooring=LoFT.Mooring, Property=LoFT.Property, Controller=LoFT.Controller, Initposition=[25,  0,  3*pi/180], Initstate=[6.8*pi/30, 9]}
      mask prompts: Aero "Aerodynamics"; Hydro "Hydrodynamics"; Mooring "Mooring lookup table"; Property "Hull mass, inertia and volume"; Controller "Local controller"; Initposition "Initial Hull position"; Initstate "Initial RotSpeed and WindEst"
      mask DialogControl DescGroupVar Prompt: LoFT
      mask DialogControl FOWT Prompt: Low-order modelling of floating offshore wind turbine for training
      mask DialogControl Manuscript Prompt: Citation
      mask DialogControl scriptname Prompt: Primary Frequency Response of Floating Offshore Wind Turbines via Deep Reinforcement Learning and Domain Randomization
      mask DialogControl ParameterGroupVar Prompt: 参数
  FOWT7 : Subsystem  mask{Aero=LoFT.Aero, Hydro=LoFT.Hydro, Mooring=LoFT.Mooring, Property=LoFT.Property, Controller=LoFT.Controller, Initposition=[15,  0,  3*pi/180], Initstate=[6.8*pi/30, 9]}
      mask prompts: Aero "Aerodynamics"; Hydro "Hydrodynamics"; Mooring "Mooring lookup table"; Property "Hull mass, inertia and volume"; Controller "Local controller"; Initposition "Initial Hull position"; Initstate "Initial RotSpeed and WindEst"
      mask DialogControl DescGroupVar Prompt: LoFT
      mask DialogControl FOWT Prompt: Low-order modelling of floating offshore wind turbine for training
      mask DialogControl Manuscript Prompt: Citation
      mask DialogControl scriptname Prompt: Primary Frequency Response of Floating Offshore Wind Turbines via Deep Reinforcement Learning and Domain Randomization
      mask DialogControl ParameterGroupVar Prompt: 参数
  FOWT8 : Subsystem  mask{Aero=LoFT.Aero, Hydro=LoFT.Hydro, Mooring=LoFT.Mooring, Property=LoFT.Property, Controller=LoFT.Controller, Initposition=[40,  0,  3*pi/180], Initstate=[6.8*pi/30, 9]}
      mask prompts: Aero "Aerodynamics"; Hydro "Hydrodynamics"; Mooring "Mooring lookup table"; Property "Hull mass, inertia and volume"; Controller "Local controller"; Initposition "Initial Hull position"; Initstate "Initial RotSpeed and WindEst"
      mask DialogControl DescGroupVar Prompt: LoFT
      mask DialogControl FOWT Prompt: Low-order modelling of floating offshore wind turbine for training
      mask DialogControl Manuscript Prompt: Citation
      mask DialogControl scriptname Prompt: Primary Frequency Response of Floating Offshore Wind Turbines via Deep Reinforcement Learning and Domain Randomization
      mask DialogControl ParameterGroupVar Prompt: 参数
  FOWT9 : Subsystem  mask{Aero=LoFT.Aero, Hydro=LoFT.Hydro, Mooring=LoFT.Mooring, Property=LoFT.Property, Controller=LoFT.Controller, Initposition=[25,  0,  3*pi/180], Initstate=[6.8*pi/30, 9]}
      mask prompts: Aero "Aerodynamics"; Hydro "Hydrodynamics"; Mooring "Mooring lookup table"; Property "Hull mass, inertia and volume"; Controller "Local controller"; Initposition "Initial Hull position"; Initstate "Initial RotSpeed and WindEst"
      mask DialogControl DescGroupVar Prompt: LoFT
      mask DialogControl FOWT Prompt: Low-order modelling of floating offshore wind turbine for training
      mask DialogControl Manuscript Prompt: Citation
      mask DialogControl scriptname Prompt: Primary Frequency Response of Floating Offshore Wind Turbines via Deep Reinforcement Learning and Domain Randomization
      mask DialogControl ParameterGroupVar Prompt: 参数
  "switch " : Subsystem
  switch 1 : Subsystem
  switch 2 : Subsystem
  switch 3 : Subsystem
  switch 4 : Subsystem
  switch 5 : Subsystem
  switch 6 : Subsystem
  switch 7 : Subsystem
  switch 8 : Subsystem
  switch 9 : Subsystem
  wave series 1 : Subsystem
  wave series 10 : Subsystem
  wave series 2 : Subsystem
  wave series 3 : Subsystem
  wave series 4 : Subsystem
  wave series 5 : Subsystem
  wave series 6 : Subsystem
  wave series 7 : Subsystem
  wave series 8 : Subsystem
  wave series 9 : Subsystem
  1 : Outport
  2 : Outport  Port=2
  3 : Outport  Port=3
  4 : Outport  Port=4
  5 : Outport  Port=5
  6 : Outport  Port=6
  7 : Outport  Port=7
  8 : Outport  Port=8
  9 : Outport  Port=9
  10 : Outport  Port=10
  wires:
  Demux/9 -> [P9]
  Demux/10 -> [P10]
  wave series 10/1(Out1) -> FOWT10/2(Waveforces)
  [B1] -> FOWT10/4(Blade Pitch(rad))
  Constant19/1 -> switch 9/1(In1)
  switch 9/1(Out1) -> FOWT10/5(Commu)
  [P10] -> FOWT10/3(Power(MW))
  [Wind10] -> FOWT10/1(Inflow wind(m/s))
  Constant11/1 -> switch 8/1(In1)
  [P9] -> FOWT9/3(Power(MW))
  [B1] -> FOWT9/4(Blade Pitch(rad))
  [Wind9] -> FOWT9/1(Inflow wind(m/s))
  switch 8/1(Out1) -> FOWT9/5(Commu)
  wave series 9/1(Out1) -> FOWT9/2(Waveforces)
  Demux/6 -> [P6]
  Demux/7 -> [P7]
  Demux/8 -> [P8]
  Demux/5 -> [P5]
  Demux/1 -> [P1]
  Demux/4 -> [P4]
  action/1 -> Demux/1
  Demux/3 -> [P3]
  Demux/2 -> [P2]
  [Wind2] -> FOWT2/1(Inflow wind(m/s))
  wave series 2/1(Out1) -> FOWT2/2(Waveforces)
  [Wind4] -> FOWT4/1(Inflow wind(m/s))
  wave series 8/1(Out1) -> FOWT8/2(Waveforces)
  [Wind3] -> FOWT3/1(Inflow wind(m/s))
  switch 4/1(Out1) -> FOWT5/5(Commu)
  switch 7/1(Out1) -> FOWT8/5(Commu)
  wave series 4/1(Out1) -> FOWT4/2(Waveforces)
  switch 6/1(Out1) -> FOWT7/5(Commu)
  Constant16/1 -> switch 7/1(In1)
  wave series 6/1(Out1) -> FOWT6/2(Waveforces)
  [Wind8] -> FOWT8/1(Inflow wind(m/s))
  wave series 1/1(Out1) -> FOWT1/2(Waveforces)
  [Wind5] -> FOWT5/1(Inflow wind(m/s))
  Constant8/1 -> "switch "/1(In1)
  "switch "/1(Out1) -> FOWT1/5(Commu)
  [P8] -> FOWT8/3(Power(MW))
  [B1] -> FOWT8/4(Blade Pitch(rad))
  wave series 5/1(Out1) -> FOWT5/2(Waveforces)
  Constant10/1 -> switch 2/1(In1)
  [P5] -> FOWT5/3(Power(MW))
  Constant14/1 -> switch 6/1(In1)
  [P6] -> FOWT6/3(Power(MW))
  Constant12/1 -> switch 5/1(In1)
  [P4] -> FOWT4/3(Power(MW))
  wave series 7/1(Out1) -> FOWT7/2(Waveforces)
  [Wind7] -> FOWT7/1(Inflow wind(m/s))
  [P1] -> FOWT1/3(Power(MW))
  [B1] -> FOWT7/4(Blade Pitch(rad))
  [P3] -> FOWT3/3(Power(MW))
  Constant1/1 -> switch 4/1(In1)
  switch 1/1(Out1) -> FOWT2/5(Commu)
  [Wind1] -> FOWT1/1(Inflow wind(m/s))
  [P2] -> FOWT2/3(Power(MW))
  [Wind6] -> FOWT6/1(Inflow wind(m/s))
  wave series 3/1(Out1) -> FOWT3/2(Waveforces)
  Constant7/1 -> switch 3/1(In1)
  Constant9/1 -> switch 1/1(In1)
  [P7] -> FOWT7/3(Power(MW))
  switch 5/1(Out1) -> FOWT6/5(Commu)
  switch 3/1(Out1) -> FOWT4/5(Commu)
  switch 2/1(Out1) -> FOWT3/5(Commu)
  Demux1/4 -> [Wind4]
  In2/1 -> Demux1/1
  Demux1/7 -> [Wind7]
  Demux1/8 -> [Wind8]
  Demux1/3 -> [Wind3]
  Demux1/2 -> [Wind2]
  Demux1/5 -> [Wind5]
  Demux1/9 -> [Wind9]
  Demux1/10 -> [Wind10]
  Demux1/1 -> [Wind1]
  Demux1/6 -> [Wind6]
  FOWT1/1(Out1) -> 1/1
  FOWT2/1(Out1) -> 2/1
  FOWT3/1(Out1) -> 3/1
  FOWT4/1(Out1) -> 4/1
  FOWT5/1(Out1) -> 5/1
  FOWT6/1(Out1) -> 6/1
  FOWT7/1(Out1) -> 7/1
  FOWT8/1(Out1) -> 8/1
  FOWT9/1(Out1) -> 9/1
  FOWT10/1(Out1) -> 10/1
  In1/1 -> [B1]
  [B1] -> FOWT1/4(Blade Pitch(rad))
  [B1] -> FOWT2/4(Blade Pitch(rad))
  [B1] -> FOWT3/4(Blade Pitch(rad))
  [B1] -> FOWT4/4(Blade Pitch(rad))
  [B1] -> FOWT5/4(Blade Pitch(rad))
  [B1] -> FOWT6/4(Blade Pitch(rad))

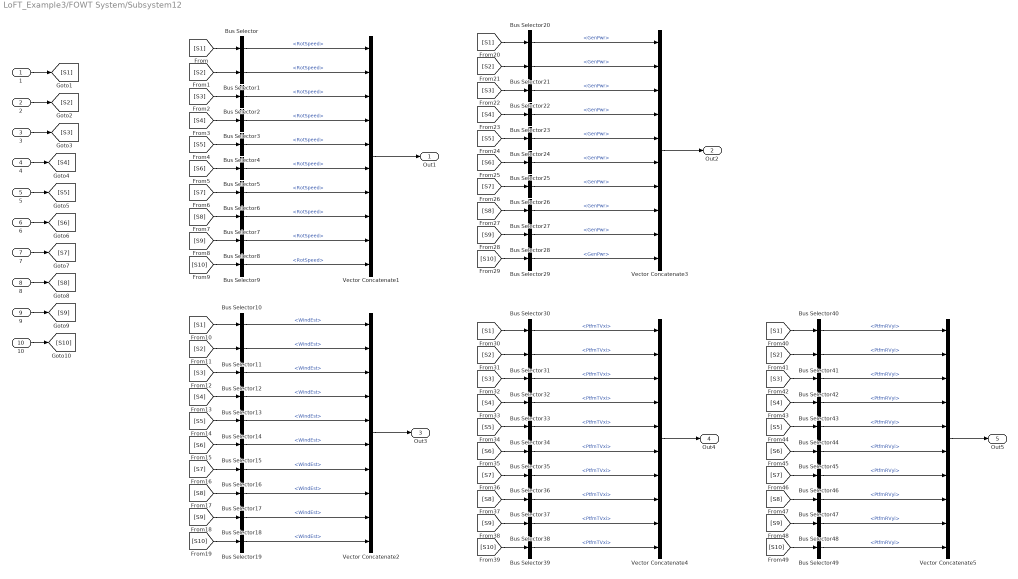
== system LoFT_Example3/FOWT System/Subsystem12 ==
  1 : Inport
  2 : Inport  Port=2
  3 : Inport  Port=3
  4 : Inport  Port=4
  5 : Inport  Port=5
  6 : Inport  Port=6
  7 : Inport  Port=7
  8 : Inport  Port=8
  9 : Inport  Port=9
  10 : Inport  Port=10
  Bus Selector{,1..9} (10 alike) : BusSelector  OutputSignals=RotSpeed
  Bus Selector{10..19} (10 alike) : BusSelector  OutputSignals=WindEst
  Bus Selector{20..29} (10 alike) : BusSelector  OutputSignals=GenPwr
  Bus Selector{30..39} (10 alike) : BusSelector  OutputSignals=PtfmTVxi
  Bus Selector{40..49} (10 alike) : BusSelector  OutputSignals=PtfmRVyi
  Vector Concatenate{1..5} (5 alike) : Concatenate  NumInputs=10
  Out1 : Outport
  Out2 : Outport  Port=2
  Out3 : Outport  Port=3
  Out4 : Outport  Port=4
  Out5 : Outport  Port=5
  wires:
  Bus Selector39/1 -> Vector Concatenate4/10  "<PtfmTVxi>"
  [S10] -> Bus Selector39/1
  Bus Selector38/1 -> Vector Concatenate4/9  "<PtfmTVxi>"
  [S9] -> Bus Selector38/1
  Bus Selector37/1 -> Vector Concatenate4/8  "<PtfmTVxi>"
  [S8] -> Bus Selector37/1
  Bus Selector36/1 -> Vector Concatenate4/7  "<PtfmTVxi>"
  [S7] -> Bus Selector36/1
  Bus Selector35/1 -> Vector Concatenate4/6  "<PtfmTVxi>"
  [S6] -> Bus Selector35/1
  Bus Selector34/1 -> Vector Concatenate4/5  "<PtfmTVxi>"
  [S5] -> Bus Selector34/1
  Bus Selector33/1 -> Vector Concatenate4/4  "<PtfmTVxi>"
  [S4] -> Bus Selector33/1
  [S3] -> Bus Selector32/1
  Bus Selector32/1 -> Vector Concatenate4/3  "<PtfmTVxi>"
  [S2] -> Bus Selector31/1
  Bus Selector31/1 -> Vector Concatenate4/2  "<PtfmTVxi>"
  [S8] -> Bus Selector47/1
  Bus Selector41/1 -> Vector Concatenate5/2  "<PtfmRVyi>"
  Bus Selector46/1 -> Vector Concatenate5/7  "<PtfmRVyi>"
  [S7] -> Bus Selector46/1
  Vector Concatenate5/1 -> Out5/1
  Bus Selector49/1 -> Vector Concatenate5/10  "<PtfmRVyi>"
  [S10] -> Bus Selector49/1
  [S6] -> Bus Selector45/1
  Bus Selector48/1 -> Vector Concatenate5/9  "<PtfmRVyi>"
  Bus Selector45/1 -> Vector Concatenate5/6  "<PtfmRVyi>"
  [S9] -> Bus Selector48/1
  Bus Selector43/1 -> Vector Concatenate5/4  "<PtfmRVyi>"
  Bus Selector44/1 -> Vector Concatenate5/5  "<PtfmRVyi>"
  Bus Selector42/1 -> Vector Concatenate5/3  "<PtfmRVyi>"
  [S3] -> Bus Selector42/1
  [S4] -> Bus Selector43/1
  [S2] -> Bus Selector41/1
  Bus Selector40/1 -> Vector Concatenate5/1  "<PtfmRVyi>"
  [S1] -> Bus Selector40/1
  Bus Selector47/1 -> Vector Concatenate5/8  "<PtfmRVyi>"
  [S5] -> Bus Selector44/1
  Vector Concatenate4/1 -> Out4/1
  Bus Selector30/1 -> Vector Concatenate4/1  "<PtfmTVxi>"
  [S1] -> Bus Selector30/1
  Vector Concatenate2/1 -> Out3/1
  Vector Concatenate3/1 -> Out2/1
  [S8] -> Bus Selector17/1
  Bus Selector29/1 -> Vector Concatenate3/10  "<GenPwr>"
  Bus Selector28/1 -> Vector Concatenate3/9  "<GenPwr>"
  Bus Selector27/1 -> Vector Concatenate3/8  "<GenPwr>"
  Bus Selector26/1 -> Vector Concatenate3/7  "<GenPwr>"
  Bus Selector25/1 -> Vector Concatenate3/6  "<GenPwr>"
  Bus Selector24/1 -> Vector Concatenate3/5  "<GenPwr>"
  [S10] -> Bus Selector29/1
  [S9] -> Bus Selector28/1
  [S8] -> Bus Selector27/1
  [S7] -> Bus Selector26/1
  [S6] -> Bus Selector25/1
  [S5] -> Bus Selector24/1
  Bus Selector23/1 -> Vector Concatenate3/4  "<GenPwr>"
  [S4] -> Bus Selector23/1
  [S3] -> Bus Selector22/1
  Bus Selector22/1 -> Vector Concatenate3/3  "<GenPwr>"
  Bus Selector21/1 -> Vector Concatenate3/2  "<GenPwr>"
  [S2] -> Bus Selector21/1
  Bus Selector20/1 -> Vector Concatenate3/1  "<GenPwr>"
  [S1] -> Bus Selector20/1
  [S1] -> Bus Selector10/1
  Bus Selector10/1 -> Vector Concatenate2/1  "<WindEst>"
  [S2] -> Bus Selector11/1
  Bus Selector11/1 -> Vector Concatenate2/2  "<WindEst>"
  Bus Selector12/1 -> Vector Concatenate2/3  "<WindEst>"
  [S3] -> Bus Selector12/1
  [S4] -> Bus Selector13/1
  Bus Selector13/1 -> Vector Concatenate2/4  "<WindEst>"
  [S5] -> Bus Selector14/1
  [S6] -> Bus Selector15/1
  [S7] -> Bus Selector16/1
  [S9] -> Bus Selector18/1
  [S10] -> Bus Selector19/1
  Bus Selector14/1 -> Vector Concatenate2/5  "<WindEst>"
  Bus Selector15/1 -> Vector Concatenate2/6  "<WindEst>"
  Bus Selector16/1 -> Vector Concatenate2/7  "<WindEst>"
  Bus Selector17/1 -> Vector Concatenate2/8  "<WindEst>"
  Bus Selector18/1 -> Vector Concatenate2/9  "<WindEst>"
  Bus Selector19/1 -> Vector Concatenate2/10  "<WindEst>"
  Bus Selector9/1 -> Vector Concatenate1/10  "<RotSpeed>"
  Bus Selector8/1 -> Vector Concatenate1/9  "<RotSpeed>"
  Bus Selector7/1 -> Vector Concatenate1/8  "<RotSpeed>"
  Bus Selector6/1 -> Vector Concatenate1/7  "<RotSpeed>"
  Bus Selector5/1 -> Vector Concatenate1/6  "<RotSpeed>"
  Bus Selector4/1 -> Vector Concatenate1/5  "<RotSpeed>"
  [S10] -> Bus Selector9/1
  [S9] -> Bus Selector8/1
  [S8] -> Bus Selector7/1
  [S7] -> Bus Selector6/1
  [S6] -> Bus Selector5/1
  [S5] -> Bus Selector4/1
  Bus Selector3/1 -> Vector Concatenate1/4  "<RotSpeed>"
  [S4] -> Bus Selector3/1
  [S3] -> Bus Selector2/1
  Bus Selector2/1 -> Vector Concatenate1/3  "<RotSpeed>"
  Bus Selector1/1 -> Vector Concatenate1/2  "<RotSpeed>"
  [S2] -> Bus Selector1/1
  Bus Selector/1 -> Vector Concatenate1/1  "<RotSpeed>"
  Vector Concatenate1/1 -> Out1/1
  [S1] -> Bus Selector/1
  10/1 -> [S10]
  9/1 -> [S9]
  8/1 -> [S8]
  7/1 -> [S7]
  6/1 -> [S6]
  5/1 -> [S5]
  4/1 -> [S4]
  3/1 -> [S3]
  2/1 -> [S2]
  1/1 -> [S1]
